simulink model "SimTrifasicoMeioLinhaComIsoladorMonofasico"  (R2022b)
settings: Solver=ode45  StartTime=0.0  StopTime=SimulacaoTempo  RelTol=1e-3  EnableMultiTasking=on
values from neighbouring files (symbols this model uses):
  C_matrix = [7.14789431755e-09  -2.14393248907e-09; -2.14393248907e-09  7.14789431755e-09]    [Modelo2fios2awg160.mat]    (also in trifasico2awg.mat = [7.86602198725e-09  -2.45195546694e-09  -1.42580481937e-09; ; trifasico2awgNew.mat = [8.93900996847e-09  -2.36457299077e-09  -1.26282974561e-09; )
  dd = [ 20 ]    [CarregaDados20km.m]
  L_matrix = [0.00251001340283  0.00125944754059; 0.00125944754059  0.00251001340283]    [Modelo2fios2awg160.mat]    (also in trifasico2awg.mat = [0.00242085814129  0.00130892171515  0.00117029227904; 0.001; trifasico2awgNew.mat = [0.0018119254645  0.000784575768319  0.000670213848675; 0.00)
  m1 = n    [CurtoCircuitos.m]    (also in CurtosComparadosMonofasicos.m)
  R_matrix = [1.15977689742  0.0576982604784; 0.0576982604784  1.15977689742]    [Modelo2fios2awg160.mat]    (also in trifasico2awg.mat = [1.15895092862  0.0568724513894  0.0568719145431; 0.05687245; trifasico2awgNew.mat = [0.213716566428  0.0989824596492  0.099050906555; 0.09898245)
  TrifTerra = ValorCurto    [CurtosComparadosMonofasicos.m]
  TrifTestA = 1e6    (= 1000000)    [CurtosComparadosMonofasicos.m]
  TrifTestB = 1e-5    (= 1e-05)    [CurtosComparadosMonofasicos.m]
  TrifTestC = 1e6    (= 1000000)    [CurtosComparadosMonofasicos.m]
undefined symbols (not defined in the file or in its folder): D11, Delta
libraries: spsSeriesRLCBranchLib x4, spsDistributedParametersLineLib x2, spsThreePhaseVIMeasurementLib x2, spsThreePhaseTransformerTwoWindingsLib x2, spsGroundLib x1, spsThreePhaseSourceLib x1, spspowerguiLib x1
settings Model: Creator=laris  LastModifiedBy=Leonardo-Felipe
settings SolverCC: AlgebraicLoopSolver=TrustRegion
settings DataIOCC: LimitDataPoints=on  SaveFormat=Array  ReturnWorkspaceOutputs=off
settings OptimizationCC: LifeSpan=inf
settings DebuggingCC: UnconnectedInputMsg=warning  UnconnectedOutputMsg=warning  UnconnectedLineMsg=warning  SFUnexpectedBacktrackingDiag=warning  SFNoUnconditionalDefaultTransitionDiag=warning  SFExecutionAtInitializationDiag=none  SFMachineParentedDataDiag=warning  ArithmeticOperatorsInVariantConditions=warning
settings HardwareCC: ProdBitPerPointer=32  ProdBitPerSizeT=32  ProdBitPerPtrDiffT=32  ProdLargestAtomicFloat=None  ProdIntDivRoundTo=Undefined  ProdEndianess=Unspecified  ProdWordSize=32  ProdHWDeviceType=32-bit Generic
settings ModelReferenceCC: EnableRefExpFcnMdlSchedulingChecks=on  PropagateSignalLabelsOutOfModel=off
settings SFSimCC: SimUseLocalCustomCode=off  CustomCodeUndefinedFunction=UseInterfaceOnly
settings RTWCC: RTWUseLocalCustomCode=off  DLArmComputeVersion=19.05
settings CodeAppCC: StateflowObjectComments=on
settings GRTTargetCC: TargetLangStandard=C89/C90 (ANSI)
settings ConfigComp: CovMetricSettings=dw  CovSaveCumulativeToWorkspaceVar=on  CovSaveSingleToWorkspaceVar=on  CovExternalEMLEnable=off
settings SimscapeCC: SimscapeNormalizeSystem=off

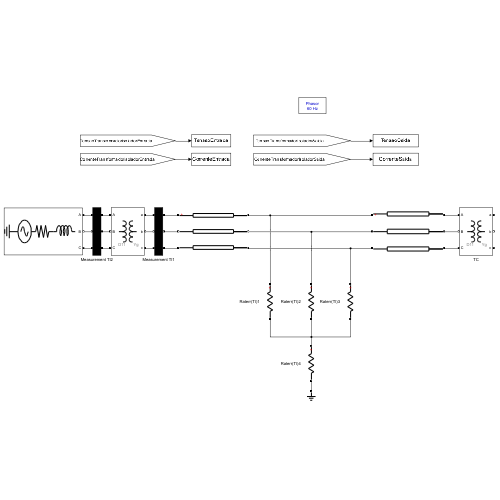
[thumbnail: Simulink's stored preview of the top-level diagram]
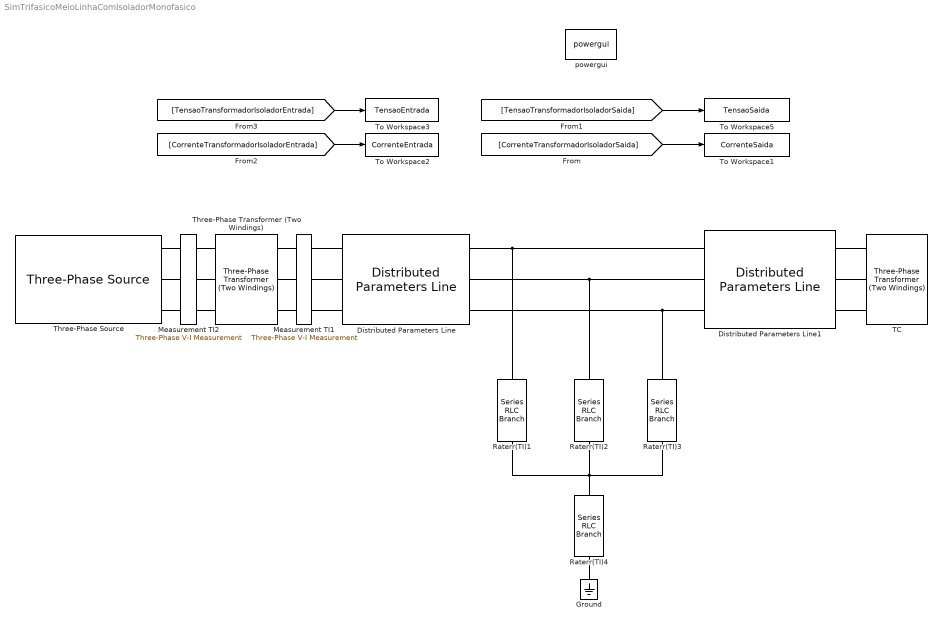
== system SimTrifasicoMeioLinhaComIsoladorMonofasico ==
  Distributed Parameters Line : spsDistributedParametersLineLib/Distributed Parameters Line  Phases=3  Length=dd * m1  Frequency=60  Resistance=R_matrix  Inductance=L_matrix  Capacitance=C_matrix  x1=[2255.3479841526 4269.75859166147 7005.6699810578;376.991118430775 376.991118430775 376.991118430775;2.70213525688193 -1.77126180696063 -2.19901725980169]  x2=[2256.38023596786 4268.99117856981 7006.05600455069;376.991118430775 376.991118430775 376.991118430775;2.70187172433276 -1.77130763945391 -2.19898043131968]  x3=[88.4359611917507 98.6317524188076 88.01668472887;376.991118430775 376.991118430775 376.991118430775;1.22988117455007 1.19757357578823 -2.02007499903288]  x4=[88.1333069487288 121.625992156637 44.4237678071261;376.991118430775 376.991118430775 376.991118430775;-1.956579228346 -1.91112293997082 1.30295983593735]  x5=2.60355177502627e-08  V1=ones(3,3)  V2=ones(3,3)  I1=ones(3,3)  I2=ones(3,3)  nHarmo=1  Measurements=None  Decoupling=on  VsMag0=[1.37261024242846 5998.96213138986 6037.14517392757]  VrMag0=[0.00311816847005049 5999.13834455791 6037.26214534615]  VsAngle0=[-72.906471310739 -138.894643293404 78.5083842107638]  VrAngle0=[-110.804364630972 -138.898906732084 78.5119946134491]  IsMag0=[156.983161529377 18.2267351972133 17.5348146125]  IrMag0=[154.503276440594 18.3175072555049 17.5281759737724]  IsAngle0=[68.1622090396034 -134.140024402079 64.5471784293276]  IrAngle0=[-109.826264221002 -125.254707466483 73.3885001709597]
  Distributed Parameters Line1 : spsDistributedParametersLineLib/Distributed Parameters Line  Phases=3  Length=dd * (1-m1)  Frequency=60  Resistance=R_matrix  Inductance=L_matrix  Capacitance=C_matrix  x1=[2256.38023596786 4268.99117856981 7006.05600455069;376.991118430775 376.991118430775 376.991118430775;2.60373976509471 -1.84839786907577 -2.27642520220176]  x2=[2267.28787590548 4281.23390056725 7026.31284305408;376.991118430775 376.991118430775 376.991118430775;2.60042511543563 -1.85533987616885 -2.28464701299214]  x3=[1.8983573882339 10.1990535711701 19.2748423912014;376.991118430775 376.991118430775 376.991118430775;2.50382525389192 -1.92872653197249 -2.35778605169105]  x4=[1.89891552635402 10.2081051937929 19.2899833243481;376.991118430775 376.991118430775 376.991118430775;2.60053115536615 -1.85562701588572 -2.28489635788094]  x5=0.000260329141984877  V1=ones(3,3)  V2=ones(3,3)  I1=ones(3,3)  I2=ones(3,3)  nHarmo=1  Measurements=None  Decoupling=on  VsMag0=[0.00311816847005049 5999.13834455791 6037.26214534615]  VrMag0=[5.45233354169978 6023.70179120883 6049.12672764814]  VsAngle0=[-110.804364630972 -138.898906732084 78.5119946134491]  VrAngle0=[-102.021503470324 -139.367197590923 78.1143644681811]  IsMag0=[2.82408223348619 17.3307827069331 16.7194854800993]  IrMag0=[2.81563274964574 17.3715213090927 16.7068396118098]  IsAngle0=[-1.53362402454544 -134.503534151176 64.5001206150892]  IrAngle0=[2.14273085380997 -130.302538561606 68.6880545857001]
  Ground : spsGroundLib/Ground  LConnTagsString=a
  Measurement TI1 : spsThreePhaseVIMeasurementLib/Three-Phase V-I Measurement  VoltageMeasurement=phase-to-phase  SetLabelV=on  LabelV=TensaoTransformadorIsoladorSaida  Vpu=off  VpuLL=off  CurrentMeasurement=yes  SetLabelI=on  LabelI=CorrenteTransformadorIsoladorSaida  Ipu=off  Pbase=100e6  Vbase=500e3  OutputType=Complex  PhasorSimulation=on  PSBequivalent=0
  Measurement TI2 : spsThreePhaseVIMeasurementLib/Three-Phase V-I Measurement  VoltageMeasurement=phase-to-phase  SetLabelV=on  LabelV=TensaoTransformadorIsoladorEntrada  Vpu=off  VpuLL=off  CurrentMeasurement=yes  SetLabelI=on  LabelI=CorrenteTransformadorIsoladorEntrada  Ipu=off  Pbase=100e6  Vbase=500e3  OutputType=Complex  PhasorSimulation=on  PSBequivalent=0
  Raterr(TI)1 : spsSeriesRLCBranchLib/Series RLC Branch  LConnTagsString=__new0  RConnTagsString=__new0  BranchType=R  Resistance=TrifTestA  Inductance=0  SetiL0=off  InitialCurrent=0  Capacitance=1e-6  Setx0=off  InitialVoltage=0  Measurements=None
  Raterr(TI)2 : spsSeriesRLCBranchLib/Series RLC Branch  LConnTagsString=__new0  RConnTagsString=__new0  BranchType=R  Resistance=TrifTestB  Inductance=0  SetiL0=off  InitialCurrent=0  Capacitance=1e-6  Setx0=off  InitialVoltage=0  Measurements=None
  Raterr(TI)3 : spsSeriesRLCBranchLib/Series RLC Branch  LConnTagsString=__new0  RConnTagsString=__new0  BranchType=R  Resistance=TrifTestC  Inductance=0  SetiL0=off  InitialCurrent=0  Capacitance=1e-6  Setx0=off  InitialVoltage=0  Measurements=None
  Raterr(TI)4 : spsSeriesRLCBranchLib/Series RLC Branch  LConnTagsString=__new0  RConnTagsString=__new0  BranchType=R  Resistance=TrifTerra  Inductance=0  SetiL0=off  InitialCurrent=0  Capacitance=1e-6  Setx0=off  InitialVoltage=0  Measurements=None
  TC : spsThreePhaseTransformerTwoWindingsLib/Three-Phase Transformer (Two Windings)  Winding1Connection=Delta (D11)  Winding2Connection=Yg  CoreType=Three single-phase transformers  SetSaturation=off  Hysteresis=off  DataFile='hysteresis'  SetInitialFlux=off  Measurements=None  UNITS=pu  NominalPower=[120e3 , 60]  Winding1=[13800 0.0048118 0.018511]  Winding2=[380 0.0048119 0.018511]  Rm=5.801193266567229e+02  Lm=8.409977380031759e+02  L0=0.50001  Saturation=[0 0;0.0012545 0.01913;0.52272 0.024231]  InitialFluxes=[0.66025 -0.66025 0.57768]  BreakLoop=off  DiscreteSolver=Trapezoidal iterative  DataType=off  TransfoNumber=1
  Three-Phase Transformer (Two Windings) : spsThreePhaseTransformerTwoWindingsLib/Three-Phase Transformer (Two Windings)  Winding1Connection=Delta (D11)  Winding2Connection=Yg  CoreType=Three single-phase transformers  SetSaturation=off  Hysteresis=off  DataFile='hysteresis'  SetInitialFlux=off  Measurements=None  UNITS=pu  NominalPower=[120e3, 60 ]  Winding1=[13800 0.004 0.023]  Winding2=[13800/sqrt(3) 0.004 0.023]  Rm=500  Lm=500  L0=0.5  Saturation=[0 0;0.0024 1.2;1 1.52]  InitialFluxes=[ 0.8 , -0.8 , 0.7 ]  BreakLoop=off  DiscreteSolver=Trapezoidal iterative  DataType=off  TransfoNumber=1
  Three-Phase Source : spsThreePhaseSourceLib/Three-Phase Source  InternalConnection=Yg  VoltagePhases=off  Voltage=13.8e3  PhaseAngle=0  Voltage_phases=[25e3 25e3 25e3]/sqrt(3)  PhaseAngles_phases=[0 -120 +120]  Frequency=60  NonIdealSource=on  SpecifyImpedance=on  Resistance=0.8929  Inductance=16.58e-3  ShortCircuitLevel=2.5e6  BaseVoltage=13.8e3  XRratio=7  BusType=swing  Pref=10e3  Qref=0  Prefabc=[10e3, 10e3, 10e3]  Qrefabc=[0, 0, 0]  Qmin=-inf  Qmax=inf
  To Workspace1 : ToWorkspace  VariableName=CorrenteSaida  SampleTime=-1
      settings: MaxDataPoints=1
  To Workspace2 : ToWorkspace  VariableName=CorrenteEntrada  SampleTime=-1
      settings: MaxDataPoints=1
  To Workspace3 : ToWorkspace  VariableName=TensaoEntrada  SampleTime=-1
      settings: MaxDataPoints=1
  To Workspace5 : ToWorkspace  VariableName=TensaoSaida  SampleTime=-1
      settings: MaxDataPoints=1
  powergui : spspowerguiLib/powergui  Priority=1  SimulationMode=Phasor  SampleTime=50e-9  frequency=60  Iterations=50  frequencyindice=60  Pbase=100e6  ErrMax=1e-4  UnitsV=kV  UnitsW=MW  buscounter=0  FunctionMessages=off  echomessages=off  EnableUseOfTLC=off  CurrentSourceSwitches=off  DisableSnubberDevices=off  DisableRonSwitches=off  DisableVfSwitches=off  DisplayEquations=off  AutomaticDiscreteSolvers=off  SolverType=Tustin/Backward Euler (TBE)  Interpol=off  ExternalGateDelay=off  methode=off  Ts=100  x0status=blocks  SPID=on  SwTol=0  HookPort=off  NonlinearTolerance=1e-4  nMaxIteration=100  ContinueOnMaxIteration=off  RestoreLinks=warning  ResistiveCurrentMeasurement=off  Frange=[0:2:500]  Ylog=off  Xlog=on  ShowGrid=off  save=off  variable=ZData  structure=0  ZoomFFT=off  StartTime=0.0  cycles=1  DisplayStyle=1  fundamental=60  FreqAxis=off  MaxFrequency=1000  frequencyindicesteady=1  RmsSteady=1  display=off
  wires:
  [CorrenteTransformadorIsoladorEntrada] -> To Workspace2/1
  [TensaoTransformadorIsoladorEntrada] -> To Workspace3/1
  [TensaoTransformadorIsoladorSaida] -> To Workspace5/1
  [CorrenteTransformadorIsoladorSaida] -> To Workspace1/1
  connections:
  Distributed Parameters Line1/LConn2 -- Raterr(TI)2/LConn1 -- Distributed Parameters Line/RConn2
  Distributed Parameters Line1/RConn1 -- TC/LConn1
  Distributed Parameters Line1/RConn2 -- TC/LConn2
  Distributed Parameters Line1/RConn3 -- TC/LConn3
  Distributed Parameters Line/LConn3 -- Measurement TI1/RConn3
  Distributed Parameters Line1/LConn3 -- Raterr(TI)3/LConn1 -- Distributed Parameters Line/RConn3
  Distributed Parameters Line/LConn1 -- Measurement TI1/RConn1
  Distributed Parameters Line/LConn2 -- Measurement TI1/RConn2
  Distributed Parameters Line1/LConn1 -- Raterr(TI)1/LConn1 -- Distributed Parameters Line/RConn1
  Three-Phase Transformer (Two Windings)/RConn1 -- Measurement TI1/LConn1
  Measurement TI1/LConn2 -- Three-Phase Transformer (Two Windings)/RConn2
  Three-Phase Transformer (Two Windings)/RConn3 -- Measurement TI1/LConn3
  Measurement TI2/RConn1 -- Three-Phase Transformer (Two Windings)/LConn1
  Measurement TI2/RConn2 -- Three-Phase Transformer (Two Windings)/LConn2
  Measurement TI2/RConn3 -- Three-Phase Transformer (Two Windings)/LConn3
  Three-Phase Source/RConn2 -- Measurement TI2/LConn2
  Three-Phase Source/RConn1 -- Measurement TI2/LConn1
  Three-Phase Source/RConn3 -- Measurement TI2/LConn3
  Raterr(TI)3/RConn1 -- Raterr(TI)2/RConn1 -- Raterr(TI)4/LConn1 -- Raterr(TI)1/RConn1
  Ground/LConn1 -- Raterr(TI)4/RConn1
